simulink model "p_controller"  (R2017b)
settings: Solver=VariableStepAuto  StartTime=0.0  StopTime=1000.0  RelTol=1e-3
settings Model: Creator=Alec  LastModifiedBy=Alec

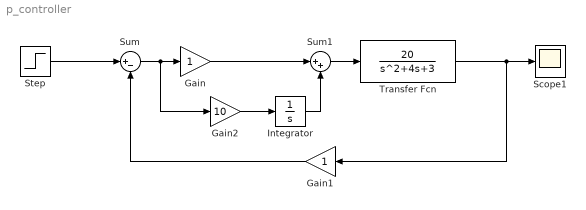
== system p_controller ==
  Gain : Gain
  Gain1 : Gain
  Gain2 : Gain  Gain=10
  Integrator : Integrator
  Scope1 : Scope
  Step : Step  SampleTime=0
  Sum : Sum  Inputs=|+-
  Sum1 : Sum  Inputs=|++
  Transfer Fcn : TransferFcn  Numerator=[20]  Denominator=[1 4 3]
  wires:
  Step/1 -> Sum/1
  Sum/1 -> Gain2/1, Gain/1
  Gain1/1 -> Sum/2
  Gain2/1 -> Integrator/1
  Sum1/1 -> Transfer Fcn/1
  Gain/1 -> Sum1/1
  Transfer Fcn/1 -> Gain1/1, Scope1/1
  Integrator/1 -> Sum1/2
